simulink model "step2"  (Simulink 7.9)
settings: Solver=ode45  StartTime=0.0  StopTime=10.0  RelTol=1e-3
values from neighbouring files (symbols this model uses):
  A = [-1.5 -0.5; -0.5 -1]    [fb_setup.m]
  P = dlyap((A+B*F)',eye(2))    [fb_setup.m]
  x0 = [1;1]    [fb_setup.m]
settings Model: Creator=aeagr  LastModifiedBy=aeagr

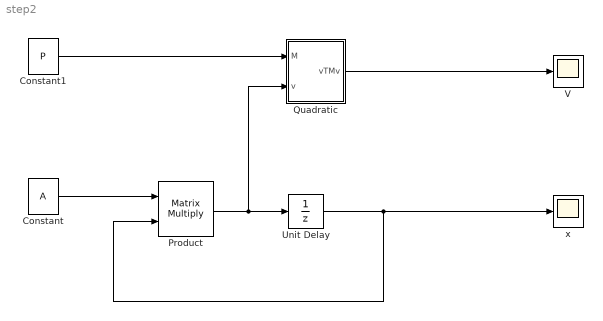
== system step2 ==
  Constant : Constant  Value=A
  Constant1 : Constant  Value=P
  Product : Product  Multiplication=Matrix(*)  RndMeth=Zero
  Quadratic : Subsystem
  Unit Delay : UnitDelay  X0=x0  SampleTime=-1
  V : Scope
  x : Scope
  wires:
  Constant/1 -> Product/1
  Product/1 -> Quadratic/2(v), Unit Delay/1
  Unit Delay/1 -> Product/2, x/1
  Constant1/1 -> Quadratic/1(M)
  Quadratic/1(vTMv) -> V/1

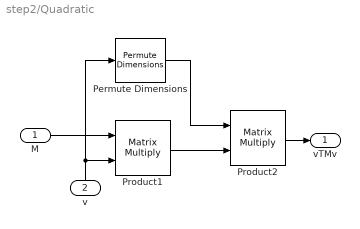
== system step2/Quadratic ==
  M : Inport
  v : Inport  Port=2
  Permute Dimensions : PermuteDimensions
  Product1 : Product  Multiplication=Matrix(*)  RndMeth=Zero
  Product2 : Product  Multiplication=Matrix(*)  RndMeth=Zero
  vTMv : Outport
  wires:
  Product1/1 -> Product2/2
  Permute Dimensions/1 -> Product2/1
  v/1 -> Product1/2, Permute Dimensions/1
  M/1 -> Product1/1
  Product2/1 -> vTMv/1
